simulink library "StateMachines"  (R2019b)
settings: Solver=VariableStepAuto  StartTime=0.0  StopTime=10.0  RelTol=1e-3  EnableMultiTasking=on
values from neighbouring files (symbols this model uses):
  Ts = ControlSampleTime    [Sim_TP3_VSM_init.m]
libraries: $bdroot x1
settings Model: Creator=cgloeckler  LastModifiedBy=e2n016
settings DataIOCC: LimitDataPoints=on  ReturnWorkspaceOutputs=off
settings OptimizationCC: LifeSpan=inf
settings DebuggingCC: AllowSymbolicDim=off  SFUnexpectedBacktrackingDiag=warning  SFNoUnconditionalDefaultTransitionDiag=warning  SFExecutionAtInitializationDiag=none  ArithmeticOperatorsInVariantConditions=warning
settings ModelReferenceCC: PropagateSignalLabelsOutOfModel=off
settings SFSimCC: SimUseLocalCustomCode=off  CustomCodeUndefinedFunction=UseInterfaceOnly
settings RTWCC: RTWUseLocalCustomCode=off
settings CodeAppCC: StateflowObjectComments=on
settings GRTTargetCC: TargetLangStandard=C89/C90 (ANSI)
settings ConfigComp: CovMetricSettings=dw  CovHtmlReporting=on  CovSaveCumulativeToWorkspaceVar=on  CovSaveSingleToWorkspaceVar=on  CovExternalEMLEnable=off

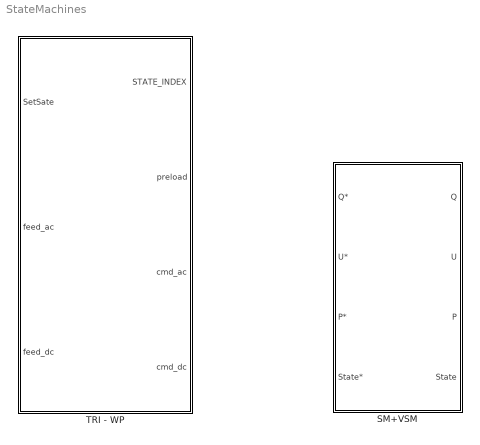
== system StateMachines ==
  SM+VSM : Subsystem  mask{Ts=0.1}
      mask prompts: Ts "Samplezeit [s]"
  TRI - WP : Subsystem  InitFcn=createTriphaseBus  mask{Time_Pre1=3, T_Pre0=3.5, T_Connect=2, T_Disconnect=0.1, T_Enable=1, T_Disable=0.1, Time_Error=5, Ts=Ts}
      mask prompts: Time_Pre1 "Time Precharge 1"; T_Pre0 "Time Precharge 0"; T_Connect "Time Connect"; T_Disconnect "Time Disconnect"; T_Enable "Time Enable Control"; T_Disable "Time Disable Control"; Time_Error "Time after Error"; Ts "Sample Time"

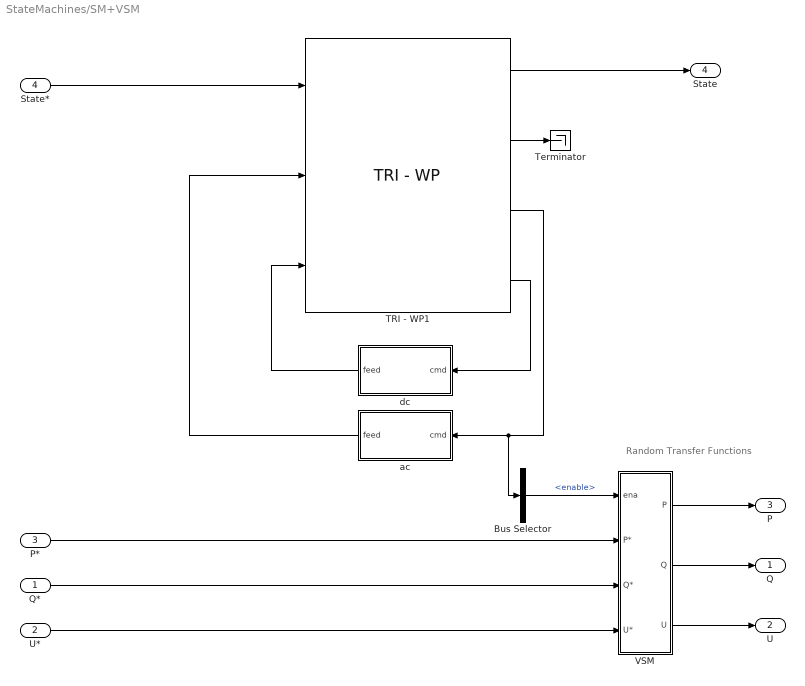
== system StateMachines/SM+VSM ==
  note: Random Transfer Functions
  Q* : Inport
  U* : Inport  Port=2
  P* : Inport  Port=3
  State* : Inport  Port=4
  Bus Selector : BusSelector  OutputSignals=enable
  TRI - WP1 : $bdroot/TRI - WP  Time_Pre1=3  T_Pre0=3.5  T_Connect=2  T_Disconnect=0.1  T_Enable=1  T_Disable=0.1  Time_Error=5  Ts=0.1
  Terminator : Terminator
  VSM : Subsystem
  ac : Subsystem
  dc : Subsystem
  Q : Outport
  U : Outport  Port=2
  P : Outport  Port=3
  State : Outport  Port=4
  wires:
  Bus Selector/1 -> VSM/1(ena)  "<enable>"
  VSM/3(U) -> U/1
  Q*/1 -> VSM/3(Q*)
  U*/1 -> VSM/4(U*)
  VSM/2(Q) -> Q/1
  VSM/1(P) -> P/1
  P*/1 -> VSM/2(P*)
  dc/1(feed) -> TRI - WP1/3
  ac/1(feed) -> TRI - WP1/2
  TRI - WP1/4 -> dc/1(cmd)
  TRI - WP1/3 -> Bus Selector/1, ac/1(cmd)
  TRI - WP1/2 -> Terminator/1
  State*/1 -> TRI - WP1/1
  TRI - WP1/1 -> State/1

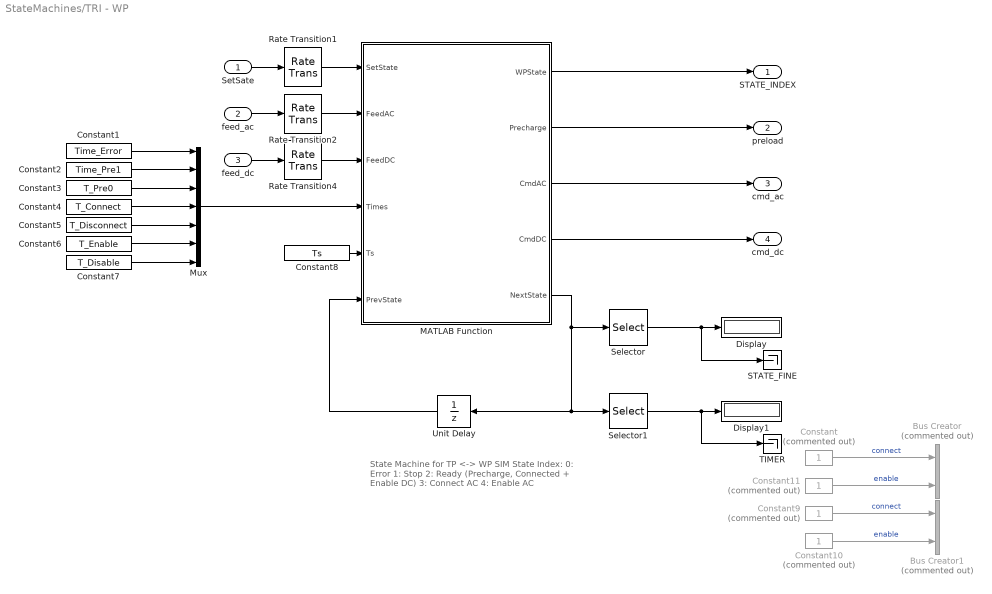
== system StateMachines/TRI - WP ==
  note: State Machine for TP <-> WP SIM
      |
      | State Index:
      | 0: Error
      | 1: Stop
      | 2: Ready (Precharge, Connected + Enable DC)
      | 3: Connect AC
      | 4: Enable AC
  SetSate : Inport
  feed_ac : Inport  Port=2
  feed_dc : Inport  Port=3
  Bus Creator : BusCreator  Commented=on  Inputs=2  OutDataTypeStr=Bus: CommandDCBus
  Bus Creator1 : BusCreator  Commented=on  Inputs=2  OutDataTypeStr=Bus: CommandACBus
  Constant{,9..11} (4 alike) : Constant  Commented=on
  Constant1 : Constant  Value=Time_Error
  Constant2 : Constant  Value=Time_Pre1
  Constant3 : Constant  Value=T_Pre0
  Constant4 : Constant  Value=T_Connect
  Constant5 : Constant  Value=T_Disconnect
  Constant6 : Constant  Value=T_Enable
  Constant7 : Constant  Value=T_Disable
  Constant8 : Constant  Value=Ts
  Display : Display
  Display1 : Display
  MATLAB Function : MATLAB Function  TreatAsAtomicUnit=on
  Mux : Mux  Inputs=7
  Rate Transition1 : RateTransition  OutPortSampleTime=Ts
  Rate Transition2 : RateTransition  OutPortSampleTime=Ts
  Rate Transition4 : RateTransition  OutPortSampleTime=Ts
  STATE_FINE : Terminator
  Selector : Selector  InputPortWidth=3  IndexOptions=Index vector (dialog)  Indices=1  OutputSizes=1
  Selector1 : Selector  InputPortWidth=3  IndexOptions=Index vector (dialog)  Indices=2  OutputSizes=1
  TIMER : Terminator
  Unit Delay : UnitDelay  InitialCondition=[1 0 0]  SampleTime=Ts  HasFrameUpgradeWarning=on
  STATE_INDEX : Outport
  preload : Outport  Port=2
  cmd_ac : Outport  Port=3
  cmd_dc : Outport  Port=4
  wires:
  MATLAB Function/4(CmdDC) -> cmd_dc/1
  MATLAB Function/3(CmdAC) -> cmd_ac/1
  Constant11/1 -> Bus Creator/2  "enable"
  Constant10/1 -> Bus Creator1/2  "enable"
  Constant9/1 -> Bus Creator1/1  "connect"
  Constant/1 -> Bus Creator/1  "connect"
  MATLAB Function/1(WPState) -> STATE_INDEX/1
  MATLAB Function/2(Precharge) -> preload/1
  Rate Transition1/1 -> MATLAB Function/1(SetState)
  Rate Transition4/1 -> MATLAB Function/3(FeedDC)
  Rate Transition2/1 -> MATLAB Function/2(FeedAC)
  Mux/1 -> MATLAB Function/4(Times)
  feed_ac/1 -> Rate Transition2/1
  feed_dc/1 -> Rate Transition4/1
  Constant7/1 -> Mux/7
  Constant6/1 -> Mux/6
  Constant5/1 -> Mux/5
  Constant4/1 -> Mux/4
  Constant3/1 -> Mux/3
  Constant2/1 -> Mux/2
  Constant1/1 -> Mux/1
  Selector1/1 -> TIMER/1, Display1/1
  Selector/1 -> Display/1, STATE_FINE/1
  MATLAB Function/5(NextState) -> Selector/1, Unit Delay/1, Selector1/1
  Unit Delay/1 -> MATLAB Function/6(PrevState)
  Constant8/1 -> MATLAB Function/5(Ts)
  SetSate/1 -> Rate Transition1/1

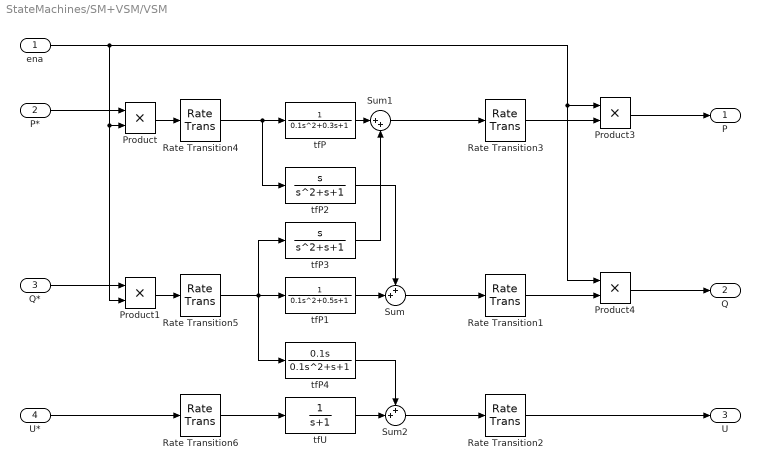
== system StateMachines/SM+VSM/VSM ==
  ena : Inport
  P* : Inport  Port=2
  Q* : Inport  Port=3
  U* : Inport  Port=4
  Product{,1,3..4} (4 alike) : Product
  Rate Transition1 : RateTransition  OutPortSampleTime=Ts
  Rate Transition2 : RateTransition  OutPortSampleTime=Ts
  Rate Transition3 : RateTransition  OutPortSampleTime=Ts
  Rate Transition4 : RateTransition
  Rate Transition5 : RateTransition
  Rate Transition6 : RateTransition
  Sum : Sum  Inputs=++|
  Sum1 : Sum  Inputs=|++
  Sum2 : Sum  Inputs=++|
  tfP : TransferFcn  Denominator=[0.1 0.3 1]
  tfP1 : TransferFcn  Denominator=[0.1 0.5 1]
  tfP2 : TransferFcn  Numerator=[1 0]  Denominator=[1 1 1]
  tfP3 : TransferFcn  Numerator=[1 0]  Denominator=[1 1 1]
  tfP4 : TransferFcn  Numerator=[0.1 0]  Denominator=[0.1 1 1]
  tfU : TransferFcn  Denominator=[1 1]
  P : Outport
  Q : Outport  Port=2
  U : Outport  Port=3
  wires:
  Rate Transition6/1 -> tfU/1
  Rate Transition5/1 -> tfP1/1, tfP3/1, tfP4/1
  Rate Transition4/1 -> tfP/1, tfP2/1
  Rate Transition2/1 -> U/1
  Rate Transition1/1 -> Product4/2
  Rate Transition3/1 -> Product3/2
  tfP4/1 -> Sum2/1
  Sum2/1 -> Rate Transition2/1
  tfU/1 -> Sum2/2
  tfP3/1 -> Sum1/2
  Sum1/1 -> Rate Transition3/1
  tfP/1 -> Sum1/1
  Sum/1 -> Rate Transition1/1
  tfP2/1 -> Sum/1
  tfP1/1 -> Sum/2
  Q*/1 -> Product1/1
  Product3/1 -> P/1
  P*/1 -> Product/1
  Product4/1 -> Q/1
  ena/1 -> Product1/2, Product/2, Product4/1, Product3/1
  U*/1 -> Rate Transition6/1
  Product1/1 -> Rate Transition5/1
  Product/1 -> Rate Transition4/1

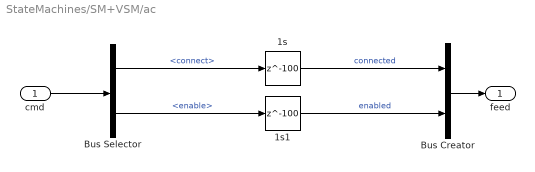
== system StateMachines/SM+VSM/ac ==
  cmd : Inport
  1s : Delay  DelayLength=100  SampleTime=Ts
  1s1 : Delay  DelayLength=100  SampleTime=Ts
  Bus Creator : BusCreator  Inputs=2  OutDataTypeStr=Bus: FeedbackACBus
  Bus Selector : BusSelector  OutputSignals=connect,enable
  feed : Outport
  wires:
  1s/1 -> Bus Creator/1  "connected"
  Bus Selector/1 -> 1s/1  "<connect>"
  Bus Selector/2 -> 1s1/1  "<enable>"
  1s1/1 -> Bus Creator/2  "enabled"
  cmd/1 -> Bus Selector/1
  Bus Creator/1 -> feed/1

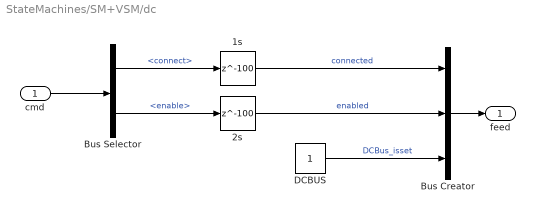
== system StateMachines/SM+VSM/dc ==
  cmd : Inport
  1s : Delay  DelayLength=100  SampleTime=Ts
  2s : Delay  DelayLength=100  SampleTime=Ts
  Bus Creator : BusCreator  Inputs=3  OutDataTypeStr=Bus: FeedbackDCBus
  Bus Selector : BusSelector  OutputSignals=connect,enable
  DCBUS : Constant
  feed : Outport
  wires:
  DCBUS/1 -> Bus Creator/3  "DCBus_isset"
  Bus Creator/1 -> feed/1
  1s/1 -> Bus Creator/1  "connected"
  cmd/1 -> Bus Selector/1
  Bus Selector/1 -> 1s/1  "<connect>"
  Bus Selector/2 -> 2s/1  "<enable>"
  2s/1 -> Bus Creator/2  "enabled"

== matlab function StateMachines/TRI - WP/MATLAB Function ==
  data: SetState input; FeedAC input; FeedDC input; Times input; Ts input; WPState output; Precharge output; CmdAC output Bus: CommandACBus =0; CmdDC output Bus: CommandDCBus =0; PrevState input; NextState output
function [WPState, Precharge, CmdAC, CmdDC, NextState] = stateMachineTriWP(SetState,FeedAC,FeedDC,Times,Ts,PrevState)
%#codegen
%Decode Memory State
NextState = PrevState;
TheState  = PrevState(1);
TheTime   = PrevState(2);
TimeSign  = PrevState(3);

%% DEFINE
STATE_ERR = 0;
STATE_OFF = 1.0;
STATE_PRE = 1.8;
STATE_CDC = 1.9;
STATE_EDC = 2.0;
STATE_CAC = 3.0;
STATE_EAC = 4.0;

TIME_ERR0 = Times(1);
TIME_PRE1 = Times(2);
TIME_PRE0 = Times(3);
TIME_CON1 = Times(4);
TIME_CON0 = Times(5);
TIME_ENA1 = Times(6);
TIME_ENA0 = Times(7);

%FEEDBACK
FB_DCcon = FeedDC.connected;
FB_DCctr = FeedDC.DCBus_isset && FeedDC.enabled;
FB_ACcon = FeedAC.connected;
FB_ACena = FeedAC.enabled;

ALL_STATES = [STATE_ERR, STATE_OFF, STATE_PRE, STATE_CDC, STATE_EDC, STATE_CAC, STATE_EAC];
All_TIMES1 = [0,         0        , TIME_PRE1, TIME_CON1, TIME_ENA1, TIME_CON1, TIME_ENA1];
All_TIMES0 = [TIME_ERR0, 0        , TIME_PRE0, TIME_CON0, TIME_ENA0, TIME_CON0  TIME_ENA0];
ALL_FEED   = [1,         1,         1,         FB_DCcon,  FB_DCctr,  FB_ACcon,  FB_ACena ];               

MIN_STATE = ALL_STATES(1);
MAX_STATE = ALL_STATES(end);
NR_STATES = length(ALL_STATES);
              %P  CA EA CD ED
TRICOMMANDS = [0  0  0  0  0;...  %STATE_ERR
               0  0  0  0  0;...  %STATE_OFF
               1  0  0  0  0;...  %STATE_PRE
               1  0  0  1  0;...  %STATE_CDC
               1  0  0  1  1;...  %STATE_EDC
               1  1  0  1  1;...  %STATE_CAC
               1  1  1  1  1];    %STATE_EAC
           

%% Check Inputs
SetState = min(max(MIN_STATE,SetState),MAX_STATE);
ISetState = find(ALL_STATES<=SetState,1,'last');
ISetState = ISetState(1);

TheState = min(max(MIN_STATE,TheState),MAX_STATE);
ITheState = find(ALL_STATES==TheState,1);
ITheState = ITheState(1);

TheTime = abs(TheTime);

if ISetState == 1 || any(ALL_FEED(1:ITheState-1) == 0)
    %Error or Feedback Gone
    INextState = 1;
    TheTime    = All_TIMES0(INextState);
    TimeSign   = 1;
elseif TheTime > 0 || ~ALL_FEED(ITheState)
    % Wait for Timer or
    % Wait for Feedback
    INextState = ITheState;
    TheTime    = TimeSign*max(TheTime - Ts,0); %Decrease Timer
    TimeSign   = sign(TimeSign); 
else
    if ISetState > ITheState
        % Go in state higher
        INextState = min(ITheState + 1,NR_STATES);
        TheTime  = All_TIMES1(INextState);
        TimeSign = +1;
    elseif ISetState < ITheState;
        % Go one state lower
        INextState = max(ITheState - 1,1);
        TheTime  = -All_TIMES0(INextState+1);
        TimeSign = -1;
    else
        INextState = ISetState;
        TheTime  = 0;
        TimeSign = 0;
    end
end

%sign(ISetState - ITheState);
TheState = ALL_STATES(INextState);
NextState(1) = TheState;
NextState(2) = TheTime;
NextState(3) = TimeSign;
%% STATE FOR WP SIM

WPState = floor(ALL_STATES(min(NR_STATES,max(1,INextState-TimeSign))));
WPState = min(max(MIN_STATE,WPState),MAX_STATE);

%% Decode Output
Precharge = TRICOMMANDS(INextState,1);
CmdAC = struct('connect', TRICOMMANDS(INextState,2), 'enable',  TRICOMMANDS(INextState,3));
CmdDC = struct('connect', TRICOMMANDS(INextState,4), 'enable',  TRICOMMANDS(INextState,5));
end
